simulink model "test_psi_cam"  (R2015a)
settings: Solver=ode45  StartTime=0.0  StopTime=inf  RelTol=1e-3
InitFcn:
  | Initilization_simulink
undefined symbols (not defined in the file): backim, drone1
libraries: visionsinks x1
settings Model: Creator=tzwijger  LastModifiedBy=tzwijger

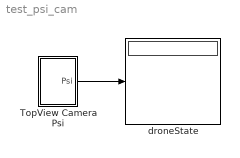
== system test_psi_cam ==
  TopView Camera Psi : Subsystem
  droneState : Display
  wires:
  TopView Camera Psi/1(Psi) -> droneState/1

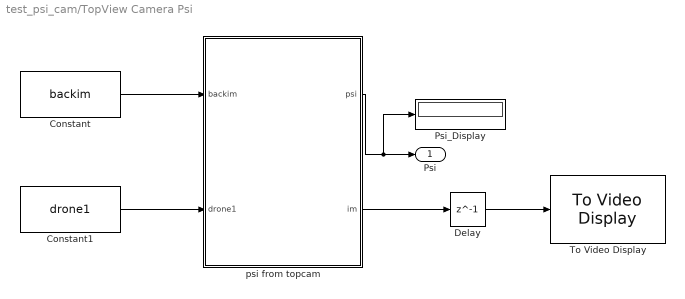
== system test_psi_cam/TopView Camera Psi ==
  Constant : Constant  Value=backim
  Constant1 : Constant  Value=drone1
  Delay : Delay  DelayLength=1  SampleTime=1/2000
  Psi_Display : Display
  To Video Display : visionsinks/To Video Display  windowSizeMode=True size (1:1)  openAtMdlStart=on  fullScreen=off  videoWindowX=40  videoWindowY=53  saveWindowSize=off  videoWindowWidth=1916  videoWindowHeight=1053  inputColorFormat=RGB  inputType=Obsolete  imagePorts=One multidimensional signal  OutputDevice=On-screen video monitor  dataOrg=Column-major  isWindowOpen=off
  psi from topcam : MATLAB Function  TreatAsAtomicUnit=on
  Psi : Outport
  wires:
  Constant1/1 -> psi from topcam/2(drone1)
  Constant/1 -> psi from topcam/1(backim)
  psi from topcam/1(psi) -> Psi_Display/1, Psi/1
  psi from topcam/2(im) -> Delay/1
  Delay/1 -> To Video Display/1

== matlab function test_psi_cam/TopView Camera Psi/psi from topcam ==
  data: backim input; psi output; drone1 input; im output
function [psi,im] = fcn(backim, drone1)
%% get psi angle from top camera
% this function is the improcdrones.m implemented for ONLY ONE DRONE and 
% therefore reduced.

coder.extrinsic('psi_topviewcam_wrapped')
    
    psi = 0;
    im = uint8(zeros(size(backim)));
    [psi,im] = psi_topviewcam_wrapped(backim, drone1);

end
